simulink model "leader_guide"  (R2022a)
settings: Solver=VariableStepAuto  StartTime=0.0  StopTime=40  RelTol=1e-3
settings Model: Creator=Column  LastModifiedBy=Column

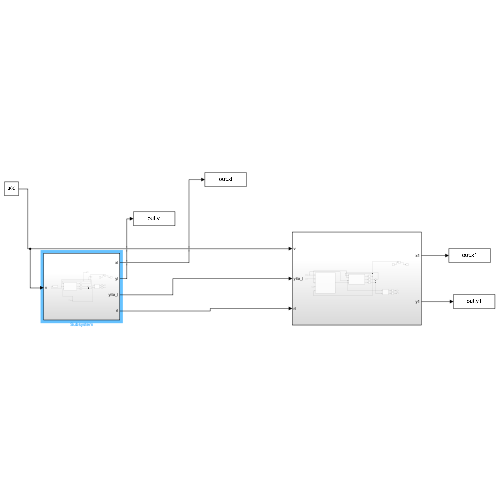
[thumbnail: Simulink's stored preview of the top-level diagram]
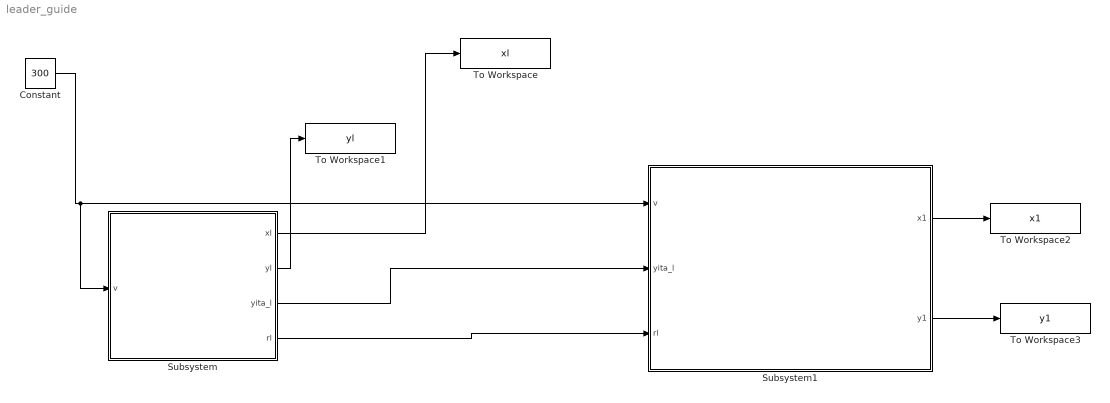
== system leader_guide ==
  Constant : Constant  Value=300
  Subsystem : Subsystem
  Subsystem1 : Subsystem
  To Workspace : ToWorkspace  VariableName=xl  SaveFormat=Timeseries  SampleTime=-1
  To Workspace1 : ToWorkspace  VariableName=yl  SaveFormat=Timeseries  SampleTime=-1
  To Workspace2 : ToWorkspace  VariableName=x1  SaveFormat=Timeseries  SampleTime=-1
  To Workspace3 : ToWorkspace  VariableName=y1  SaveFormat=Timeseries  SampleTime=-1
  wires:
  Constant/1 -> Subsystem1/1(v), Subsystem/1(v)
  Subsystem/3(yita_l) -> Subsystem1/2(yita_l)
  Subsystem/4(rl) -> Subsystem1/3(rl)
  Subsystem/1(xl) -> To Workspace/1
  Subsystem/2(yl) -> To Workspace1/1
  Subsystem1/1(x1) -> To Workspace2/1
  Subsystem1/2(y1) -> To Workspace3/1

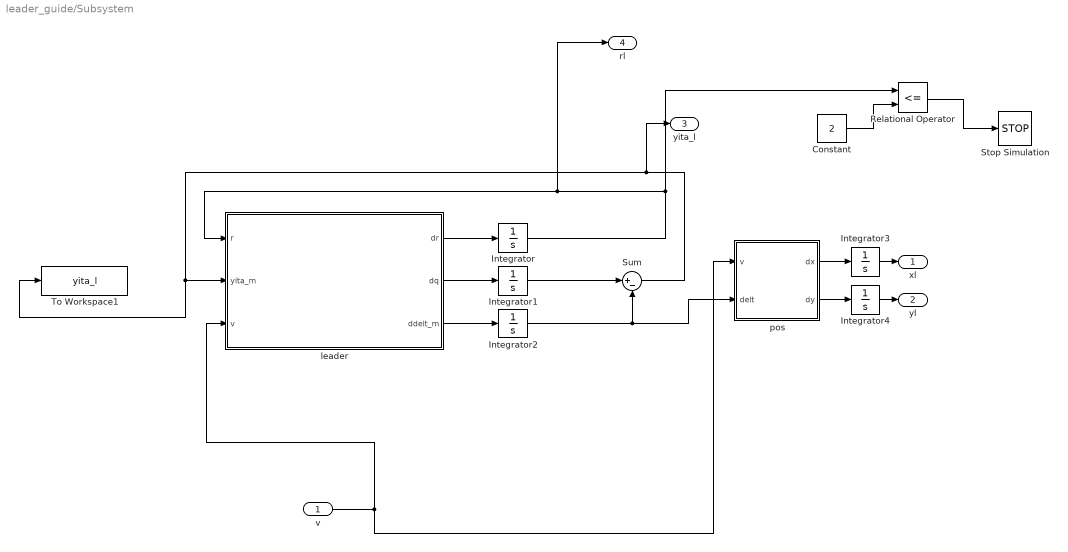
== system leader_guide/Subsystem ==
  v : Inport
  Constant : Constant  Value=2
  Integrator : Integrator  InitialCondition=sqrt(9093^2 + 5250^2)
  Integrator1 : Integrator  InitialCondition=-30 / 180 * pi
  Integrator2 : Integrator  InitialCondition=-40 * pi / 180
  Integrator3 : Integrator  InitialCondition=-9093
  Integrator4 : Integrator  InitialCondition=5250
  Relational Operator : RelationalOperator  Operator=<=  OutDataTypeStr=boolean  RndMeth=Simplest  InputSameDT=off
  Stop Simulation : Stop
  Sum : Sum  Inputs=|+-
  To Workspace1 : ToWorkspace  VariableName=yita_l  SaveFormat=Timeseries  SampleTime=-1
  leader : MATLAB Function  TreatAsAtomicUnit=on
  pos : MATLAB Function  TreatAsAtomicUnit=on
  xl : Outport
  yl : Outport  Port=2
  yita_l : Outport  Port=3
  rl : Outport  Port=4
  wires:
  Integrator3/1 -> xl/1
  pos/2(dy) -> Integrator4/1
  leader/3(ddelt_m) -> Integrator2/1
  leader/2(dq) -> Integrator1/1
  Integrator4/1 -> yl/1
  Integrator/1 -> Relational Operator/1, rl/1, leader/1(r)
  Sum/1 -> yita_l/1, To Workspace1/1, leader/2(yita_m)
  leader/1(dr) -> Integrator/1
  Integrator2/1 -> pos/2(delt), Sum/2
  Integrator1/1 -> Sum/1
  pos/1(dx) -> Integrator3/1
  v/1 -> pos/1(v), leader/3(v)
  Constant/1 -> Relational Operator/2
  Relational Operator/1 -> Stop Simulation/1

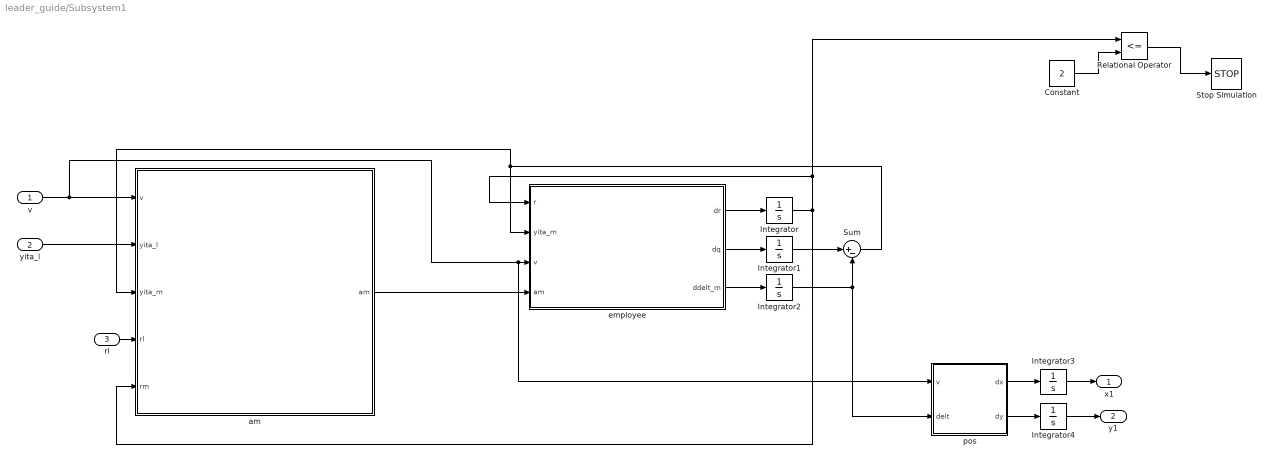
== system leader_guide/Subsystem1 ==
  v : Inport
  yita_l : Inport  Port=2
  rl : Inport  Port=3
  Constant : Constant  Value=2
  Integrator : Integrator  InitialCondition=sqrt(4750^2 + 8227^2)
  Integrator1 : Integrator  InitialCondition=120 * pi / 180
  Integrator2 : Integrator  InitialCondition=105 * pi / 180
  Integrator3 : Integrator  InitialCondition=4750
  Integrator4 : Integrator  InitialCondition=-8227
  Relational Operator : RelationalOperator  Operator=<=  OutDataTypeStr=boolean  RndMeth=Simplest  InputSameDT=off
  Stop Simulation : Stop
  Sum : Sum  Inputs=|+-
  am : MATLAB Function  TreatAsAtomicUnit=on
  employee : MATLAB Function  TreatAsAtomicUnit=on
  pos : MATLAB Function  TreatAsAtomicUnit=on
  x1 : Outport
  y1 : Outport  Port=2
  wires:
  v/1 -> pos/1(v), employee/3(v), am/1(v)
  Integrator1/1 -> Sum/1
  employee/3(ddelt_m) -> Integrator2/1
  Sum/1 -> employee/2(yita_m), am/3(yita_m)
  Integrator2/1 -> pos/2(delt), Sum/2
  employee/2(dq) -> Integrator1/1
  employee/1(dr) -> Integrator/1
  am/1(am) -> employee/4(am)
  yita_l/1 -> am/2(yita_l)
  rl/1 -> am/4(rl)
  pos/1(dx) -> Integrator3/1
  Integrator3/1 -> x1/1
  pos/2(dy) -> Integrator4/1
  Integrator4/1 -> y1/1
  Constant/1 -> Relational Operator/2
  Relational Operator/1 -> Stop Simulation/1
  Integrator/1 -> am/5(rm), Relational Operator/1, employee/1(r)

== matlab function leader_guide/Subsystem/pos ==
  data: v input; dx output; delt input; dy output
function [dx,dy] = fcn(v,delt)

dx = v * cos(delt);

dy = v * sin(delt);

== matlab function leader_guide/Subsystem/leader ==
  data: r input; yita_m input; v input; dr output; dq output; ddelt_m output
function [dr,dq,ddelt_m] = fcn(r,yita_m,v)


n = 3;


dr = -v * cos(yita_m);

dq = (v * sin(yita_m))/r;


ddelt_m = n * dq ;

== matlab function leader_guide/Subsystem1/employee ==
  data: r input; yita_m input; v input; dr output; dq output; ddelt_m output; am input
function [dr,dq,ddelt_m] = fcn(r,yita_m,v,am)


n = 3;

dr = -v * cos(yita_m);

dq = (v * sin(yita_m))/r;


ddelt_m = n * dq + am/v ;

== matlab function leader_guide/Subsystem1/am ==
  data: v input; yita_l input; yita_m input; am output; rl input; rm input
function am  = fcn(v,yita_l,yita_m,rl,rm)

n = 3;


e_yita = yita_l - yita_m;

e_r = rl - rm;

c1 = 0.7;
c2 = 0.9;


kr = c1 / (c2 + (e_r/v));

k_yita = 5;






tmp_t1 = sin(yita_l - e_yita) / (rl - e_r);


tt = cos(yita_l) - kr * e_r / v ;

if(abs(tt) > 1)
disp(tt);
disp(yita_l);
disp(e_r);
disp(kr);
disp(rl);
end

tmp_t2 = (sin(yita_l))^2 / ( rl * sqrt( 1 - (cos(yita_l) - kr * e_r / v)^2 ) ); 

t1 = -(n-1)*v^2*(tmp_t1 - tmp_t2);

t2 = ( kr^2 * e_r ) / sqrt( 1 - (cos(yita_l) - kr * e_r / v)^2 );


t3 = k_yita * v * (e_yita - yita_l + acos(cos(yita_l) - kr * e_r / v));

am = t1 + t2 - t3;


end

== matlab function leader_guide/Subsystem1/pos ==
  data: v input; dx output; delt input; dy output
function [dx,dy] = fcn(v,delt)

dx = v * cos(delt);

dy = v * sin(delt);
